simulink model "HW5_1"  (R2016a)
settings: Solver=VariableStepAuto  StartTime=0.0  StopTime=10  RelTol=1e-3
settings Model: Creator=Teng-Hu  LastModifiedBy=Teng-Hu
settings GRTTargetCC: GeneratePreprocessorConditionals=Use local settings

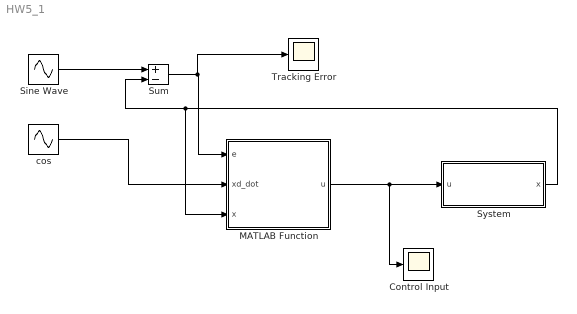
== system HW5_1 ==
  Control Input : Scope
  MATLAB Function : MATLAB Function  TreatAsAtomicUnit=on
  Sine Wave : Sin  SampleTime=0
  Sum : Sum  Inputs=+-
  System : Subsystem
  Tracking Error : Scope
  "cos " : Sin  Phase=pi/2  SampleTime=0
  wires:
  MATLAB Function/1(u) -> Control Input/1, System/1(u)
  Sine Wave/1 -> Sum/1
  System/1(x) -> MATLAB Function/3(x), Sum/2
  Sum/1 -> Tracking Error/1, MATLAB Function/1(e)
  "cos "/1 -> MATLAB Function/2(xd_dot)

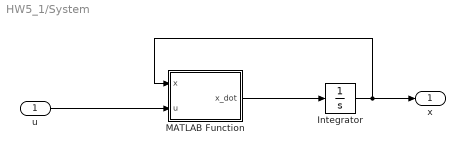
== system HW5_1/System ==
  u : Inport
  Integrator : Integrator  InitialCondition=1
  MATLAB Function : MATLAB Function  TreatAsAtomicUnit=on
  x : Outport
  wires:
  MATLAB Function/1(x_dot) -> Integrator/1
  Integrator/1 -> MATLAB Function/1(x), x/1
  u/1 -> MATLAB Function/2(u)

== matlab function HW5_1/MATLAB Function ==
  data: e input; u output; xd_dot input; x input
function u = fcn(e,xd_dot,x)
%#codegen
a=2;
b=5;
k=5;
u = xd_dot+k*e-(a*x+b*cos(x));

== matlab function HW5_1/System/MATLAB Function ==
  data: x input; u input; x_dot output
function x_dot = fcn(x,u)
%#codegen

x_dot = 2*x+5*cos(x)+u;
